simulink model "untitled_2021a"  (R2021a)
settings: Solver=VariableStepAuto  StartTime=0.0  StopTime=inf  RelTol=1e-3
undefined symbols (not defined in the file or in its folder): DiscIntNeverNeededParam
libraries: mobileRoboticsLib x17
settings Model: Creator=its_ghani  LastModifiedBy=nitis

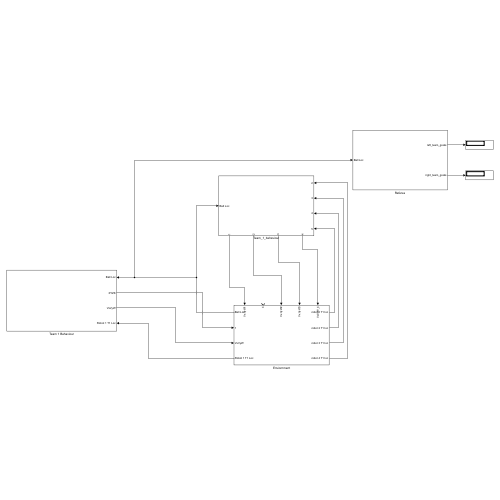
[thumbnail: Simulink's stored preview of the top-level diagram]
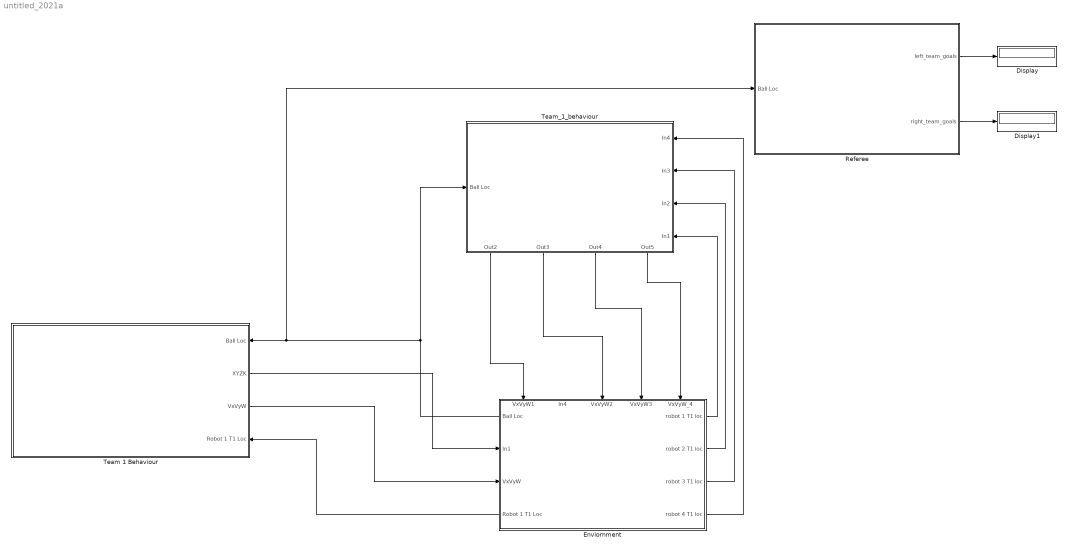
== system untitled_2021a ==
  Display : Display
  Display1 : Display
  Enviornment : Subsystem
      settings: PortSchema="{\"entries\":[{\"content\":{\"sides\":[{\"content\":{\"connectorIds\":[\"Out5\",\"In1\",\"In2\",\"Out6\"]},\"type\":\"ConnectorPlacement.EquallySpacedRectSide\",\"uuid\":\"bfc4f995-18bb-40a5-813e-439d500b4bf9\"},{\"content\":{\"connectorIds\":[\"Out1\",\"Out2\",\"Out3\",\"Out4\"],\"side\":\"RIGHT\"},\"type\":\"ConnectorPlacement.EquallySpacedRectSide\",\"uuid\":\"3fb6b8a6-16df-4a59-8ba5-6321e26d1fdd\"},{\"content\":{\"connectorIds\":[\"In3\",\"In4\",\"In5\",\"In6\",\"In7\"],\"side\":\"TOP\"},\"type\":\"ConnectorPlacement.EquallySpacedRectSide\",\"uuid\":\"a9e4cd1b-3afe-4395-99fa-15aef12a4070\"}]},\"type\":\"ConnectorPlacement.EquallySpacedConnector\",\"uuid\":\"a6ca697e-fe67-43ac-b669-91f3e6c836c9\"}],\"packageUris\":[\"http://schema.mathworks.com/mf0/Connector/R2020b\"],\"version\":\"1.0\"}"
  Referee : Subsystem
  Team 1 Behaviour : Subsystem
      settings: PortSchema="{\"entries\":[{\"content\":{\"sides\":[{\"content\":{\"connectorIds\":[]},\"type\":\"ConnectorPlacement.EquallySpacedRectSide\",\"uuid\":\"be901545-21b9-45e5-bac5-a8cb9027aef5\"},{\"content\":{\"connectorIds\":[\"In1\",\"Out1\",\"Out2\",\"In2\"],\"side\":\"RIGHT\"},\"type\":\"ConnectorPlacement.EquallySpacedRectSide\",\"uuid\":\"b7c1eb84-2f14-4c7f-a74c-d56efbe0743e\"},{\"content\":{\"connectorIds\":[],\"side\":\"TOP\"},\"type\":\"ConnectorPlacement.EquallySpacedRectSide\",\"uuid\":\"aca41723-ed3f-4bd2-8fc1-457d075e3460\"}]},\"type\":\"ConnectorPlacement.EquallySpacedConnector\",\"uuid\":\"e10e22f1-c8f0-4dfc-85d2-4ba01528372d\"}],\"packageUris\":[\"http://schema.mathworks.com/mf0/Connector/R2020b\"],\"version\":\"1.0\"}"
  Team_1_behaviour : Subsystem
      settings: PortSchema="{\"entries\":[{\"content\":{\"sides\":[{\"content\":{\"connectorIds\":[\"In1\"]},\"type\":\"ConnectorPlacement.EquallySpacedRectSide\",\"uuid\":\"3d238569-03e8-47ba-93af-d09e13fdb2d4\"},{\"content\":{\"connectorIds\":[\"In2\",\"In3\",\"In4\",\"In5\"],\"side\":\"RIGHT\"},\"type\":\"ConnectorPlacement.EquallySpacedRectSide\",\"uuid\":\"12d8afb4-4727-4f82-8566-507ab080c6de\"},{\"content\":{\"connectorIds\":[],\"side\":\"TOP\"},\"type\":\"ConnectorPlacement.EquallySpacedRectSide\",\"uuid\":\"c52fa7ec-51b7-43be-84ca-6ce417c012c7\"},{\"content\":{\"connectorIds\":[\"Out1\",\"Out2\",\"Out3\",\"Out4\"],\"side\":\"BOTTOM\"},\"type\":\"ConnectorPlacement.EquallySpacedRectSide\",\"uuid\":\"1ba4ac49-8e90-4b3f-8374-c14756940453\"}]},\"type\":\"ConnectorPlacement.EquallySpacedConnector\",\"uuid\":\"883bb5df-d6b2-498f-94a4-3b94e28c6a8f\"}],\"packageUris\":[\"http://schema.mathworks.com/mf0/Connector/R2020b\"],\"version\":\"1.0\"}"
  wires:
  Enviornment/5(Ball Loc) -> Team_1_behaviour/1(Ball Loc), Referee/1(Ball Loc), Team 1 Behaviour/1(Ball Loc)
  Team 1 Behaviour/1(XYZK) -> Enviornment/1(In1)
  Referee/2(right_team_goals) -> Display1/1
  Referee/1(left_team_goals) -> Display/1
  Team 1 Behaviour/2(VxVyW) -> Enviornment/2(VxVyW)
  Enviornment/6(Robot 1 T1 Loc) -> Team 1 Behaviour/2(Robot 1 T1 Loc)
  Team_1_behaviour/1(Out2) -> Enviornment/3(VxVyW1)
  Team_1_behaviour/2(Out3) -> Enviornment/5(VxVyW2)
  Team_1_behaviour/3(Out4) -> Enviornment/6(VxVyW3)
  Team_1_behaviour/4(Out5) -> Enviornment/7(VxVyW_4)
  Enviornment/1(robot 1 T1 loc) -> Team_1_behaviour/5(In1)
  Enviornment/2(robot 2 T1 loc) -> Team_1_behaviour/4(In2)
  Enviornment/3(robot 3 T1 loc) -> Team_1_behaviour/3(In3)
  Enviornment/4(robot 4 T1 loc) -> Team_1_behaviour/2(In4)

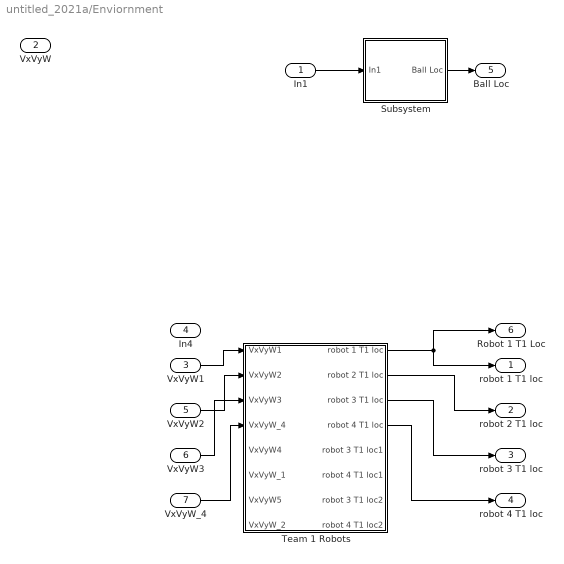
== system untitled_2021a/Enviornment ==
  In1 : Inport
  VxVyW : Inport  Port=2
  VxVyW1 : Inport  Port=3
  In4 : Inport  Port=4
  VxVyW2 : Inport  Port=5
  VxVyW3 : Inport  Port=6
  VxVyW_4 : Inport  Port=7
  "\tTeam 1 Robots" : Subsystem
  Subsystem : Subsystem
  robot 1 T1 loc : Outport
  robot 2 T1 loc : Outport  Port=2
  robot 3 T1 loc : Outport  Port=3
  robot 4 T1 loc : Outport  Port=4
  Ball Loc : Outport  Port=5
  Robot 1 T1 Loc : Outport  Port=6
  wires:
  "\tTeam 1 Robots"/1(robot 1 T1 loc) -> robot 1 T1 loc/1, Robot 1 T1 Loc/1
  "\tTeam 1 Robots"/2(robot 2 T1 loc) -> robot 2 T1 loc/1
  "\tTeam 1 Robots"/3(robot 3 T1 loc) -> robot 3 T1 loc/1
  "\tTeam 1 Robots"/4(robot 4 T1 loc) -> robot 4 T1 loc/1
  VxVyW1/1 -> "\tTeam 1 Robots"/1(VxVyW1)
  VxVyW2/1 -> "\tTeam 1 Robots"/2(VxVyW2)
  VxVyW3/1 -> "\tTeam 1 Robots"/3(VxVyW3)
  VxVyW_4/1 -> "\tTeam 1 Robots"/4(VxVyW_4)
  In1/1 -> Subsystem/1(In1)
  Subsystem/1(Ball Loc) -> Ball Loc/1

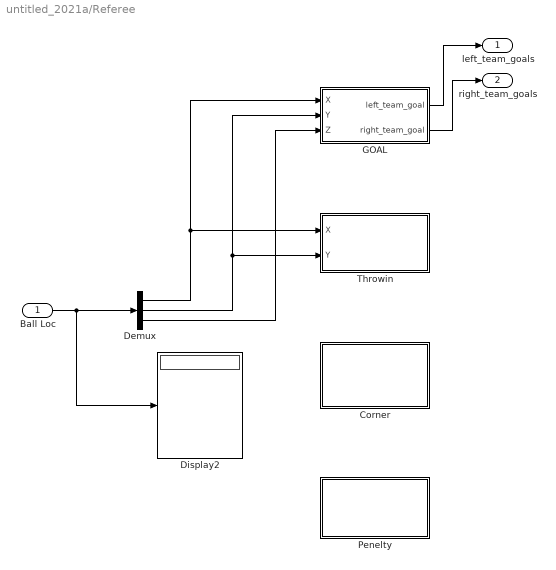
== system untitled_2021a/Referee ==
  Ball Loc : Inport
  Corner : Stateflow chart  TreatAsAtomicUnit=on
  Demux : Demux  Outputs=3
  Display2 : Display
  GOAL : Stateflow chart  TreatAsAtomicUnit=on
  Penelty : Stateflow chart  TreatAsAtomicUnit=on
  Throwin : Stateflow chart  TreatAsAtomicUnit=on
  left_team_goals : Outport
  right_team_goals : Outport  Port=2
  wires:
  Ball Loc/1 -> Display2/1, Demux/1
  Demux/1 -> Throwin/1(X), GOAL/1(X)
  Demux/2 -> Throwin/2(Y), GOAL/2(Y)
  Demux/3 -> GOAL/3(Z)
  GOAL/1(left_team_goal) -> left_team_goals/1
  GOAL/2(right_team_goal) -> right_team_goals/1

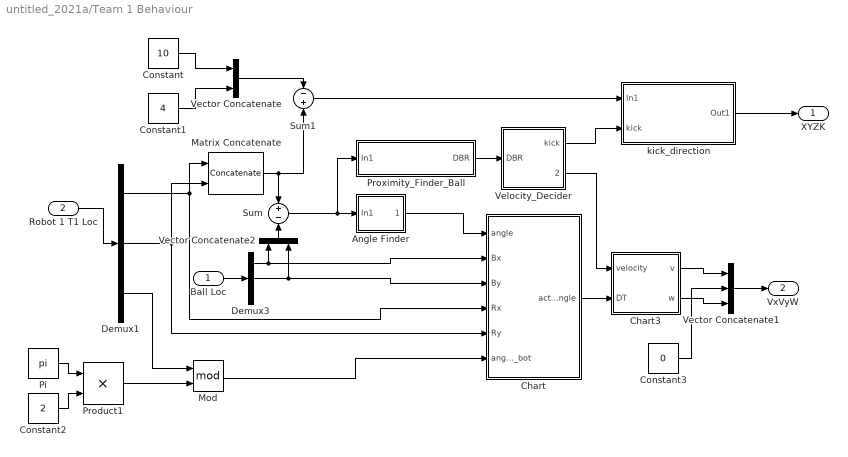
== system untitled_2021a/Team 1 Behaviour ==
  Ball Loc : Inport
  Robot 1 T1 Loc : Inport  Port=2
  Angle Finder : Subsystem
  Chart : Stateflow chart  TreatAsAtomicUnit=on
      settings: PortSchema="{\"entries\":[{\"content\":{\"sides\":[{\"content\":{\"connectorIds\":[\"In5\",\"In1\",\"In2\",\"In3\",\"In4\",\"In6\"]},\"type\":\"ConnectorPlacement.EquallySpacedRectSide\",\"uuid\":\"cd25ea97-6441-4246-83f2-eec847899c89\"},{\"content\":{\"connectorIds\":[\"Out1\"],\"side\":\"RIGHT\"},\"type\":\"ConnectorPlacement.EquallySpacedRectSide\",\"uuid\":\"ef7d77a7-1549-4474-8b84-35bb8af5d0e7\"},{\"content\":{\"connectorIds\":[],\"side\":\"TOP\"},\"type\":\"ConnectorPlacement.EquallySpacedRectSide\",\"uuid\":\"0f0ce596-3061-42ac-890a-62bc4f21ac3e\"},{\"content\":{\"connectorIds\":[],\"side\":\"BOTTOM\"},\"type\":\"ConnectorPlacement.EquallySpacedRectSide\",\"uuid\":\"682b3de5-e999-4954-b7ff-f16ecbf9ea8f\"}]},\"type\":\"ConnectorPlacement.EquallySpacedConnector\",\"uuid\":\"15dca8e2-6a60-4a0d-80a5-3c295a61c828\"}],\"packageUris\":[\"http://schema.mathworks.com/mf0/Connector/R2020b\"],\"version\":\"1.0\"}"
  Chart3 : Stateflow chart  TreatAsAtomicUnit=on
  Constant : Constant  Value=10
  Constant1 : Constant  Value=4
  Constant2 : Constant  Value=2
  Constant3 : Constant  Value=0
  Demux1 : Demux  Outputs=3
  Demux3 : Demux  Outputs=3
  Matrix Concatenate : Concatenate  Mode=Multidimensional array  ConcatenateDimension=2
  Mod : Math  Operator=mod  SaturateOnIntegerOverflow=on
  Pi : Constant  Value=pi  OutDataTypeStr=Inherit: Inherit via back propagation
  Product1 : Product
  Proximity_Finder_Ball : Subsystem
  Sum : Sum  Inputs=+-
  Sum1 : Sum  Inputs=-+
  Vector Concatenate : Concatenate
  Vector Concatenate1 : Concatenate  NumInputs=3
  Vector Concatenate2 : Concatenate
  Velocity_Decider : Stateflow chart  TreatAsAtomicUnit=on
  kick_direction : Subsystem
  XYZK : Outport
  VxVyW : Outport  Port=2
  wires:
  Ball Loc/1 -> Demux3/1
  Sum/1 -> Proximity_Finder_Ball/1(In1), Angle Finder/1(In1)
  Robot 1 T1 Loc/1 -> Demux1/1
  Demux1/1 -> Matrix Concatenate/1, Chart/3(Rx)
  Demux1/2 -> Matrix Concatenate/2, Chart/4(Ry)
  Matrix Concatenate/1 -> Sum1/2, Sum/1
  Demux3/2 -> Vector Concatenate2/2, Chart/2(By)
  Demux3/1 -> Vector Concatenate2/1, Chart/1(Bx)
  Demux1/3 -> Mod/1
  Pi/1 -> Product1/1
  Constant2/1 -> Product1/2
  Product1/1 -> Mod/2
  Chart/1(actual_angle) -> Chart3/2(DT)
  Mod/1 -> Chart/6(angle_bot)
  Angle Finder/1(angle) -> Chart/5(angle)
  Proximity_Finder_Ball/1(DBR) -> Velocity_Decider/1(DBR)
  Velocity_Decider/2(velocity) -> Chart3/1(velocity)
  Constant/1 -> Vector Concatenate/1
  Constant1/1 -> Vector Concatenate/2
  Vector Concatenate/1 -> Sum1/1
  Sum1/1 -> kick_direction/1(In1)
  Velocity_Decider/1(kick) -> kick_direction/2(kick)
  kick_direction/1(Out1) -> XYZK/1
  Chart3/1(v) -> Vector Concatenate1/1
  Chart3/2(w) -> Vector Concatenate1/3
  Constant3/1 -> Vector Concatenate1/2
  Vector Concatenate1/1 -> VxVyW/1
  Vector Concatenate2/1 -> Sum/2

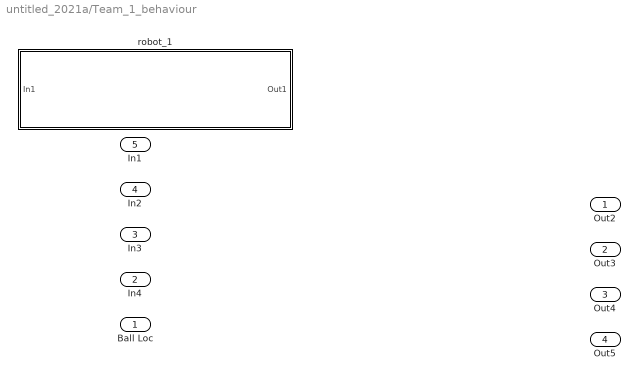
== system untitled_2021a/Team_1_behaviour ==
  Ball Loc : Inport
  In4 : Inport  Port=2
  In3 : Inport  Port=3
  In2 : Inport  Port=4
  In1 : Inport  Port=5
  robot_1 : Subsystem
  Out2 : Outport
  Out3 : Outport  Port=2
  Out4 : Outport  Port=3
  Out5 : Outport  Port=4

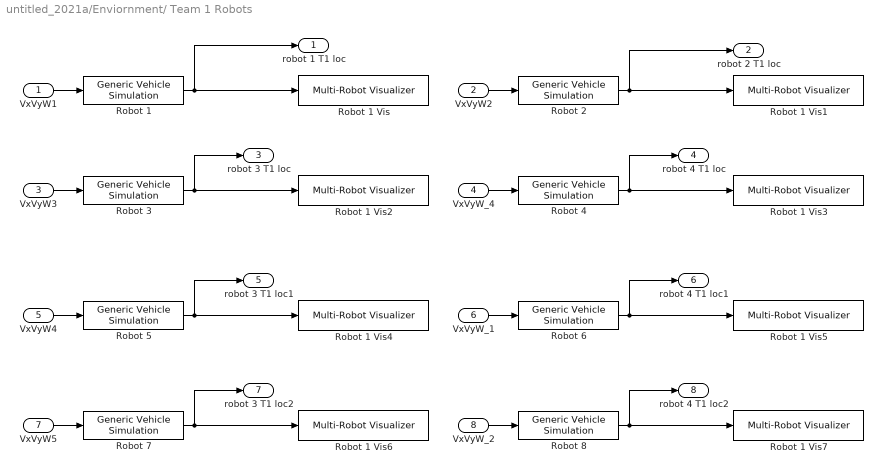
== system untitled_2021a/Enviornment/	Team 1 Robots ==
  VxVyW1 : Inport
  VxVyW2 : Inport  Port=2
  VxVyW3 : Inport  Port=3
  VxVyW_4 : Inport  Port=4
  VxVyW4 : Inport  Port=5
  VxVyW_1 : Inport  Port=6
  VxVyW5 : Inport  Port=7
  VxVyW_2 : Inport  Port=8
  Robot 1 : mobileRoboticsLib/Utilities/Generic Vehicle Simulation  initX=1.5  initY=4  initAngle=0  Ts=0.05
      settings: SourceProductName=Mobile Robotics Simulation Toolbox
  Robot 1 Vis : mobileRoboticsLib/Environments/Multi-Robot Visualizer  idx=1  radius=0.311/2  robotColor=[0 0 1]  showTraj=on  hasLidar=off  sensorOffset=[0,0]  scanAngles=[-pi/4, 0, pi/4]  maxNumScans=0  hasObjDetector=off  objDetectorOffset=[0,0]  objDetectorAngle=0  objDetectorFOV=pi/3  objDetectorMaxRange=5  hasRobotDetector=off  robotDetectorOffset=[0,0]  robotDetectorAngle=0  robotDetectorFOV=pi/3  robotDetectorMaxRange=5  robotDetectorNumDetections=0
      settings: SourceProductName=Mobile Robotics Simulation Toolbox
  Robot 1 Vis1 : mobileRoboticsLib/Environments/Multi-Robot Visualizer  idx=2  radius=0.311/2  robotColor=[0 0 1]  showTraj=on  hasLidar=off  sensorOffset=[0,0]  scanAngles=[-pi/4, 0, pi/4]  maxNumScans=0  hasObjDetector=off  objDetectorOffset=[0,0]  objDetectorAngle=0  objDetectorFOV=pi/3  objDetectorMaxRange=5  hasRobotDetector=off  robotDetectorOffset=[0,0]  robotDetectorAngle=0  robotDetectorFOV=pi/3  robotDetectorMaxRange=5  robotDetectorNumDetections=0
      settings: SourceProductName=Mobile Robotics Simulation Toolbox
  Robot 1 Vis2 : mobileRoboticsLib/Environments/Multi-Robot Visualizer  idx=3  radius=0.311/2  robotColor=[0 0 1]  showTraj=on  hasLidar=off  sensorOffset=[0,0]  scanAngles=[-pi/4, 0, pi/4]  maxNumScans=0  hasObjDetector=off  objDetectorOffset=[0,0]  objDetectorAngle=0  objDetectorFOV=pi/3  objDetectorMaxRange=5  hasRobotDetector=off  robotDetectorOffset=[0,0]  robotDetectorAngle=0  robotDetectorFOV=pi/3  robotDetectorMaxRange=5  robotDetectorNumDetections=0
      settings: SourceProductName=Mobile Robotics Simulation Toolbox
  Robot 1 Vis3 : mobileRoboticsLib/Environments/Multi-Robot Visualizer  idx=4  radius=0.311/2  robotColor=[0 0 1]  showTraj=on  hasLidar=off  sensorOffset=[0,0]  scanAngles=[-pi/4, 0, pi/4]  maxNumScans=0  hasObjDetector=off  objDetectorOffset=[0,0]  objDetectorAngle=0  objDetectorFOV=pi/3  objDetectorMaxRange=5  hasRobotDetector=off  robotDetectorOffset=[0,0]  robotDetectorAngle=0  robotDetectorFOV=pi/3  robotDetectorMaxRange=5  robotDetectorNumDetections=0
      settings: SourceProductName=Mobile Robotics Simulation Toolbox
  Robot 1 Vis4 : mobileRoboticsLib/Environments/Multi-Robot Visualizer  idx=5  radius=0.311/2  robotColor=[1 0 0]  showTraj=on  hasLidar=off  sensorOffset=[0,0]  scanAngles=[-pi/4, 0, pi/4]  maxNumScans=0  hasObjDetector=off  objDetectorOffset=[0,0]  objDetectorAngle=0  objDetectorFOV=pi/3  objDetectorMaxRange=5  hasRobotDetector=off  robotDetectorOffset=[0,0]  robotDetectorAngle=0  robotDetectorFOV=pi/3  robotDetectorMaxRange=5  robotDetectorNumDetections=0
      settings: SourceProductName=Mobile Robotics Simulation Toolbox
  Robot 1 Vis5 : mobileRoboticsLib/Environments/Multi-Robot Visualizer  idx=6  radius=0.311/2  robotColor=[1 0 0]  showTraj=on  hasLidar=off  sensorOffset=[0,0]  scanAngles=[-pi/4, 0, pi/4]  maxNumScans=0  hasObjDetector=off  objDetectorOffset=[0,0]  objDetectorAngle=0  objDetectorFOV=pi/3  objDetectorMaxRange=5  hasRobotDetector=off  robotDetectorOffset=[0,0]  robotDetectorAngle=0  robotDetectorFOV=pi/3  robotDetectorMaxRange=5  robotDetectorNumDetections=0
      settings: SourceProductName=Mobile Robotics Simulation Toolbox
  Robot 1 Vis6 : mobileRoboticsLib/Environments/Multi-Robot Visualizer  idx=7  radius=0.311/2  robotColor=[1 0 0]  showTraj=on  hasLidar=off  sensorOffset=[0,0]  scanAngles=[-pi/4, 0, pi/4]  maxNumScans=0  hasObjDetector=off  objDetectorOffset=[0,0]  objDetectorAngle=0  objDetectorFOV=pi/3  objDetectorMaxRange=5  hasRobotDetector=off  robotDetectorOffset=[0,0]  robotDetectorAngle=0  robotDetectorFOV=pi/3  robotDetectorMaxRange=5  robotDetectorNumDetections=0
      settings: SourceProductName=Mobile Robotics Simulation Toolbox
  Robot 1 Vis7 : mobileRoboticsLib/Environments/Multi-Robot Visualizer  idx=8  radius=0.311/2  robotColor=[1 0 0]  showTraj=on  hasLidar=off  sensorOffset=[0,0]  scanAngles=[-pi/4, 0, pi/4]  maxNumScans=0  hasObjDetector=off  objDetectorOffset=[0,0]  objDetectorAngle=0  objDetectorFOV=pi/3  objDetectorMaxRange=5  hasRobotDetector=off  robotDetectorOffset=[0,0]  robotDetectorAngle=0  robotDetectorFOV=pi/3  robotDetectorMaxRange=5  robotDetectorNumDetections=0
      settings: SourceProductName=Mobile Robotics Simulation Toolbox
  Robot 2 : mobileRoboticsLib/Utilities/Generic Vehicle Simulation  initX=3.25  initY=2.5  initAngle=0  Ts=0.05
      settings: SourceProductName=Mobile Robotics Simulation Toolbox
  Robot 3 : mobileRoboticsLib/Utilities/Generic Vehicle Simulation  initX=3.25  initY=5.5  initAngle=0  Ts=0.05
      settings: SourceProductName=Mobile Robotics Simulation Toolbox
  Robot 4 : mobileRoboticsLib/Utilities/Generic Vehicle Simulation  initX=5.25  initY=4.25  initAngle=0  Ts=0.05
      settings: SourceProductName=Mobile Robotics Simulation Toolbox
  Robot 5 : mobileRoboticsLib/Utilities/Generic Vehicle Simulation  initX=9.5  initY=4  initAngle=pi  Ts=0.05
      settings: SourceProductName=Mobile Robotics Simulation Toolbox
  Robot 6 : mobileRoboticsLib/Utilities/Generic Vehicle Simulation  initX=7.75  initY=4  initAngle=pi  Ts=0.05
      settings: SourceProductName=Mobile Robotics Simulation Toolbox
  Robot 7 : mobileRoboticsLib/Utilities/Generic Vehicle Simulation  initX=7.75  initY=5.5  initAngle=pi  Ts=0.05
      settings: SourceProductName=Mobile Robotics Simulation Toolbox
  Robot 8 : mobileRoboticsLib/Utilities/Generic Vehicle Simulation  initX=7.75  initY=2.5  initAngle=pi  Ts=0.05
      settings: SourceProductName=Mobile Robotics Simulation Toolbox
  robot 1 T1 loc : Outport
  robot 2 T1 loc : Outport  Port=2
  robot 3 T1 loc : Outport  Port=3
  robot 4 T1 loc : Outport  Port=4
  robot 3 T1 loc1 : Outport  Port=5
  robot 4 T1 loc1 : Outport  Port=6
  robot 3 T1 loc2 : Outport  Port=7
  robot 4 T1 loc2 : Outport  Port=8
  wires:
  Robot 1/1 -> robot 1 T1 loc/1, Robot 1 Vis/1
  VxVyW1/1 -> Robot 1/1
  VxVyW2/1 -> Robot 2/1
  Robot 2/1 -> robot 2 T1 loc/1, Robot 1 Vis1/1
  Robot 3/1 -> Robot 1 Vis2/1, robot 3 T1 loc/1
  VxVyW3/1 -> Robot 3/1
  VxVyW_4/1 -> Robot 4/1
  Robot 4/1 -> robot 4 T1 loc/1, Robot 1 Vis3/1
  VxVyW4/1 -> Robot 5/1
  Robot 5/1 -> robot 3 T1 loc1/1, Robot 1 Vis4/1
  Robot 6/1 -> Robot 1 Vis5/1, robot 4 T1 loc1/1
  VxVyW_1/1 -> Robot 6/1
  Robot 7/1 -> Robot 1 Vis6/1, robot 3 T1 loc2/1
  VxVyW5/1 -> Robot 7/1
  VxVyW_2/1 -> Robot 8/1
  Robot 8/1 -> robot 4 T1 loc2/1, Robot 1 Vis7/1

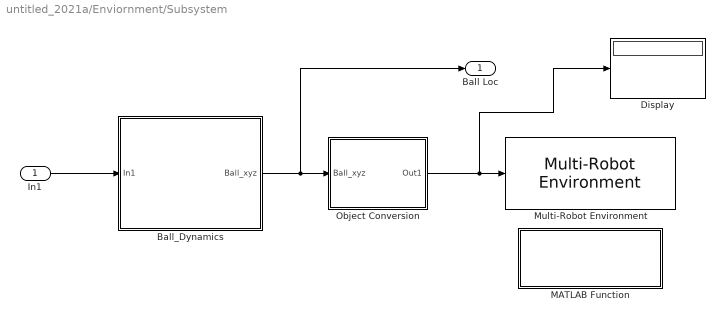
== system untitled_2021a/Enviornment/Subsystem ==
  In1 : Inport
  Ball_Dynamics : Subsystem
  Display : Display
  MATLAB Function : MATLAB Function  TreatAsAtomicUnit=on
  Multi-Robot Environment : mobileRoboticsLib/Environments/Multi-Robot Environment  numRobots=8  showWaypoints=off  showObjects=on  objectColors=[1 0 0]  objectMarkers='C'  showRobotIds=on  plotSensorLines=on
      settings: SourceProductName=Mobile Robotics Simulation Toolbox
  Object Conversion : Subsystem
  Ball Loc : Outport
  wires:
  Object Conversion/1(Out1) -> Multi-Robot Environment/1, Display/1
  Ball_Dynamics/1(Ball_xyz) -> Ball Loc/1, Object Conversion/1(Ball_xyz)
  In1/1 -> Ball_Dynamics/1(In1)

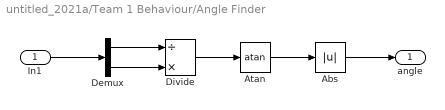
== system untitled_2021a/Team 1 Behaviour/Angle Finder ==
  In1 : Inport
  Abs : Abs
  Atan : Trigonometry  Operator=atan
  Demux : Demux  Outputs=2
  Divide : Product  Inputs=/*
  angle : Outport
  wires:
  Divide/1 -> Atan/1
  Demux/2 -> Divide/2
  Demux/1 -> Divide/1
  Atan/1 -> Abs/1
  Abs/1 -> angle/1
  In1/1 -> Demux/1

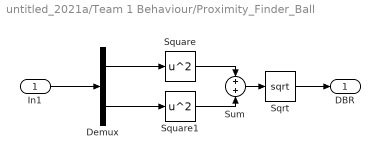
== system untitled_2021a/Team 1 Behaviour/Proximity_Finder_Ball ==
  In1 : Inport
  Demux : Demux  Outputs=2
  Sqrt : Sqrt  SaturateOnIntegerOverflow=on
  Square : Math  Operator=square  SaturateOnIntegerOverflow=on
  Square1 : Math  Operator=square  SaturateOnIntegerOverflow=on
  Sum : Sum
  DBR : Outport
  wires:
  In1/1 -> Demux/1
  Demux/1 -> Square/1
  Demux/2 -> Square1/1
  Square1/1 -> Sum/2
  Square/1 -> Sum/1
  Sum/1 -> Sqrt/1
  Sqrt/1 -> DBR/1

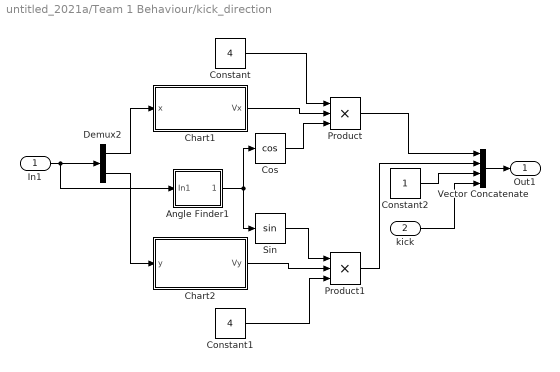
== system untitled_2021a/Team 1 Behaviour/kick_direction ==
  In1 : Inport
  kick : Inport  Port=2
  Angle Finder1 : Subsystem
  Chart1 : Stateflow chart  TreatAsAtomicUnit=on
  Chart2 : Stateflow chart  TreatAsAtomicUnit=on
  Constant : Constant  Value=4
  Constant1 : Constant  Value=4
  Constant2 : Constant
  Cos : Trigonometry  Operator=cos
  Demux2 : Demux  Outputs=2
  Product : Product  Inputs=3
  Product1 : Product  Inputs=3
  Sin : Trigonometry
  Vector Concatenate : Concatenate  NumInputs=4
  Out1 : Outport
  wires:
  Demux2/2 -> Chart2/1(y)
  Demux2/1 -> Chart1/1(x)
  In1/1 -> Angle Finder1/1(In1), Demux2/1
  Chart1/1(Vx) -> Product/2
  Cos/1 -> Product/3
  Angle Finder1/1(angle) -> Cos/1, Sin/1
  Constant/1 -> Product/1
  Constant1/1 -> Product1/3
  Chart2/1(Vy) -> Product1/2
  Sin/1 -> Product1/1
  Product/1 -> Vector Concatenate/1
  Product1/1 -> Vector Concatenate/2
  Constant2/1 -> Vector Concatenate/3
  kick/1 -> Vector Concatenate/4
  Vector Concatenate/1 -> Out1/1

== system untitled_2021a/Team_1_behaviour/robot_1 ==
  In1 : Inport
  Out1 : Outport
  wires:
  In1/1 -> Out1/1

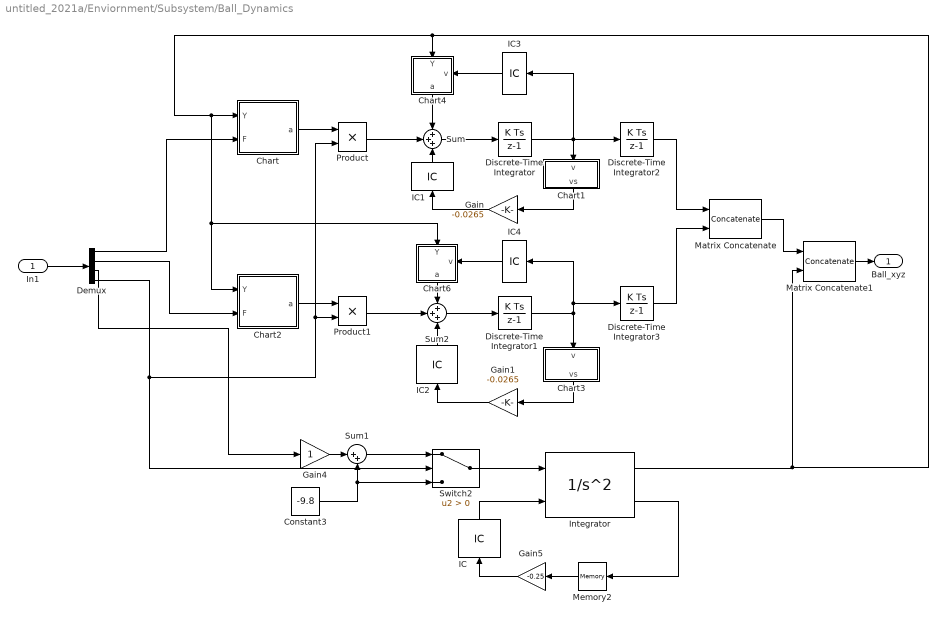
== system untitled_2021a/Enviornment/Subsystem/Ball_Dynamics ==
  In1 : Inport
  Chart : Stateflow chart  TreatAsAtomicUnit=on
  Chart1 : Stateflow chart  TreatAsAtomicUnit=on
      settings: PortSchema="{\"entries\":[{\"content\":{\"sides\":[{\"content\":{\"connectorIds\":[]},\"type\":\"ConnectorPlacement.EquallySpacedRectSide\",\"uuid\":\"edcb69b6-c92b-474e-86d7-1e52c2e82b28\"},{\"content\":{\"connectorIds\":[],\"side\":\"RIGHT\"},\"type\":\"ConnectorPlacement.EquallySpacedRectSide\",\"uuid\":\"df9771e4-6870-4305-9c84-3f71fcb76e6b\"},{\"content\":{\"connectorIds\":[\"In1\"],\"side\":\"TOP\"},\"type\":\"ConnectorPlacement.EquallySpacedRectSide\",\"uuid\":\"56b80241-156d-4669-9174-884a577f2013\"},{\"content\":{\"connectorIds\":[\"Out1\"],\"side\":\"BOTTOM\"},\"type\":\"ConnectorPlacement.EquallySpacedRectSide\",\"uuid\":\"179af6a7-cab5-4faa-a562-268e2d2e4d3e\"}]},\"type\":\"ConnectorPlacement.EquallySpacedConnector\",\"uuid\":\"707001f1-02b8-4f5e-ba3f-f155c99072e5\"}],\"packageUris\":[\"http://schema.mathworks.com/mf0/Connector/R2020b\"],\"version\":\"1.0\"}"
  Chart2 : Stateflow chart  TreatAsAtomicUnit=on
  Chart3 : Stateflow chart  TreatAsAtomicUnit=on
      settings: PortSchema="{\"entries\":[{\"content\":{\"sides\":[{\"content\":{\"connectorIds\":[]},\"type\":\"ConnectorPlacement.EquallySpacedRectSide\",\"uuid\":\"edcb69b6-c92b-474e-86d7-1e52c2e82b28\"},{\"content\":{\"connectorIds\":[],\"side\":\"RIGHT\"},\"type\":\"ConnectorPlacement.EquallySpacedRectSide\",\"uuid\":\"df9771e4-6870-4305-9c84-3f71fcb76e6b\"},{\"content\":{\"connectorIds\":[\"In1\"],\"side\":\"TOP\"},\"type\":\"ConnectorPlacement.EquallySpacedRectSide\",\"uuid\":\"56b80241-156d-4669-9174-884a577f2013\"},{\"content\":{\"connectorIds\":[\"Out1\"],\"side\":\"BOTTOM\"},\"type\":\"ConnectorPlacement.EquallySpacedRectSide\",\"uuid\":\"179af6a7-cab5-4faa-a562-268e2d2e4d3e\"}]},\"type\":\"ConnectorPlacement.EquallySpacedConnector\",\"uuid\":\"707001f1-02b8-4f5e-ba3f-f155c99072e5\"}],\"packageUris\":[\"http://schema.mathworks.com/mf0/Connector/R2020b\"],\"version\":\"1.0\"}"
  Chart4 : Stateflow chart  TreatAsAtomicUnit=on
      settings: PortSchema="{\"entries\":[{\"content\":{\"sides\":[{\"content\":{\"connectorIds\":[]},\"type\":\"ConnectorPlacement.EquallySpacedRectSide\",\"uuid\":\"edcb69b6-c92b-474e-86d7-1e52c2e82b28\"},{\"content\":{\"connectorIds\":[\"In2\"],\"side\":\"RIGHT\"},\"type\":\"ConnectorPlacement.EquallySpacedRectSide\",\"uuid\":\"df9771e4-6870-4305-9c84-3f71fcb76e6b\"},{\"content\":{\"connectorIds\":[\"In1\"],\"side\":\"TOP\"},\"type\":\"ConnectorPlacement.EquallySpacedRectSide\",\"uuid\":\"56b80241-156d-4669-9174-884a577f2013\"},{\"content\":{\"connectorIds\":[\"Out1\"],\"side\":\"BOTTOM\"},\"type\":\"ConnectorPlacement.EquallySpacedRectSide\",\"uuid\":\"6d9abc99-74e1-40c2-a49f-e0d9410a29cc\"}]},\"type\":\"ConnectorPlacement.EquallySpacedConnector\",\"uuid\":\"707001f1-02b8-4f5e-ba3f-f155c99072e5\"}],\"packageUris\":[\"http://schema.mathworks.com/mf0/Connector/R2020b\"],\"version\":\"1.0\"}"
  Chart6 : Stateflow chart  TreatAsAtomicUnit=on
      settings: PortSchema="{\"entries\":[{\"content\":{\"sides\":[{\"content\":{\"connectorIds\":[]},\"type\":\"ConnectorPlacement.EquallySpacedRectSide\",\"uuid\":\"edcb69b6-c92b-474e-86d7-1e52c2e82b28\"},{\"content\":{\"connectorIds\":[\"In2\"],\"side\":\"RIGHT\"},\"type\":\"ConnectorPlacement.EquallySpacedRectSide\",\"uuid\":\"df9771e4-6870-4305-9c84-3f71fcb76e6b\"},{\"content\":{\"connectorIds\":[\"In1\"],\"side\":\"TOP\"},\"type\":\"ConnectorPlacement.EquallySpacedRectSide\",\"uuid\":\"56b80241-156d-4669-9174-884a577f2013\"},{\"content\":{\"connectorIds\":[\"Out1\"],\"side\":\"BOTTOM\"},\"type\":\"ConnectorPlacement.EquallySpacedRectSide\",\"uuid\":\"6d9abc99-74e1-40c2-a49f-e0d9410a29cc\"}]},\"type\":\"ConnectorPlacement.EquallySpacedConnector\",\"uuid\":\"707001f1-02b8-4f5e-ba3f-f155c99072e5\"}],\"packageUris\":[\"http://schema.mathworks.com/mf0/Connector/R2020b\"],\"version\":\"1.0\"}"
  Constant3 : Constant  Value=-9.8
  Demux : Demux
  Discrete-Time Integrator : DiscreteIntegrator  SampleTime=-1  ICPrevOutput=DiscIntNeverNeededParam  ICPrevScaledInput=DiscIntNeverNeededParam
  Discrete-Time Integrator1 : DiscreteIntegrator  SampleTime=-1  ICPrevOutput=DiscIntNeverNeededParam  ICPrevScaledInput=DiscIntNeverNeededParam
  Discrete-Time Integrator2 : DiscreteIntegrator  InitialCondition=5.5  SampleTime=-1  ICPrevOutput=DiscIntNeverNeededParam  ICPrevScaledInput=DiscIntNeverNeededParam
  Discrete-Time Integrator3 : DiscreteIntegrator  InitialCondition=4  SampleTime=-1  ICPrevOutput=DiscIntNeverNeededParam  ICPrevScaledInput=DiscIntNeverNeededParam
  Gain : Gain  Gain=-0.0265
  Gain1 : Gain  Gain=-0.0265
  Gain4 : Gain
  Gain5 : Gain  Gain=-0.25
  IC : InitialCondition
  IC{1..4} (4 alike) : InitialCondition  Value=0
  Integrator : SecondOrderIntegrator  ICX=0  LimitX=on  LowerLimitX=0.0  StateNameX='Position'  ICSourceDXDT=external  StateNameDXDT='Velocity'  ReinitDXDTwhenXreachesSaturation=on
  Matrix Concatenate : Concatenate  Mode=Multidimensional array  ConcatenateDimension=2
  Matrix Concatenate1 : Concatenate  Mode=Multidimensional array  ConcatenateDimension=2
  Memory2 : Memory
  Product : Product
  Product1 : Product
  Sum : Sum  Inputs=+++
  Sum1 : Sum  Inputs=|++
  Sum2 : Sum  Inputs=+++
  Switch2 : Switch  Criteria=u2 > Threshold
  Ball_xyz : Outport
  wires:
  Constant3/1 -> Sum1/2, Switch2/3
  Integrator/2 -> Memory2/1
  Memory2/1 -> Gain5/1
  IC/1 -> Integrator/2
  Switch2/1 -> Integrator/1
  Sum1/1 -> Switch2/1
  Gain4/1 -> Sum1/1
  Matrix Concatenate/1 -> Matrix Concatenate1/1
  Matrix Concatenate1/1 -> Ball_xyz/1
  Demux/3 -> Gain4/1
  Demux/4 -> Switch2/2, Product/2, Product1/2
  Gain5/1 -> IC/1
  In1/1 -> Demux/1
  Gain/1 -> IC1/1
  Chart/1(a) -> Product/1
  Sum/1 -> Discrete-Time Integrator/1
  Discrete-Time Integrator1/1 -> IC4/1, Discrete-Time Integrator3/1, Chart3/1(v)
  Chart2/1(a) -> Product1/1
  Gain1/1 -> IC2/1
  Product1/1 -> Sum2/2
  Sum2/1 -> Discrete-Time Integrator1/1
  Demux/1 -> Chart/2(F)
  Demux/2 -> Chart2/2(F)
  Discrete-Time Integrator2/1 -> Matrix Concatenate/1
  Discrete-Time Integrator3/1 -> Matrix Concatenate/2
  Integrator/1 -> Chart6/1(Y), Chart2/1(Y), Chart/1(Y), Chart4/1(Y), Matrix Concatenate1/2
  Chart1/1(vs) -> Gain/1
  Chart3/1(vs) -> Gain1/1
  IC3/1 -> Chart4/2(v)
  Discrete-Time Integrator/1 -> IC3/1, Discrete-Time Integrator2/1, Chart1/1(v)
  Product/1 -> Sum/2
  IC2/1 -> Sum2/3
  IC1/1 -> Sum/3
  IC4/1 -> Chart6/2(v)
  Chart4/1(a) -> Sum/1
  Chart6/1(a) -> Sum2/1

== system untitled_2021a/Enviornment/Subsystem/Object Conversion ==
  Ball_xyz : Inport
  Constant : Constant
  Demux : Demux  Outputs=3
  Matrix Concatenate : Concatenate  NumInputs=3  Mode=Multidimensional array
  Out1 : Outport
  wires:
  Ball_xyz/1 -> Demux/1
  Matrix Concatenate/1 -> Out1/1
  Demux/1 -> Matrix Concatenate/1
  Demux/2 -> Matrix Concatenate/2
  Constant/1 -> Matrix Concatenate/3

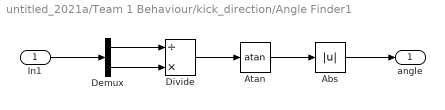
== system untitled_2021a/Team 1 Behaviour/kick_direction/Angle Finder1 ==
  In1 : Inport
  Abs : Abs
  Atan : Trigonometry  Operator=atan
  Demux : Demux  Outputs=2
  Divide : Product  Inputs=/*
  angle : Outport
  wires:
  Divide/1 -> Atan/1
  Demux/2 -> Divide/2
  Demux/1 -> Divide/1
  Atan/1 -> Abs/1
  Abs/1 -> angle/1
  In1/1 -> Demux/1

== stateflow chart untitled_2021a/Referee/Throwin ==
  data: X input; Y input

== stateflow chart untitled_2021a/Referee/Corner ==

== stateflow chart untitled_2021a/Referee/Penelty ==

== matlab function untitled_2021a/Enviornment/Subsystem/MATLAB Function ==

function plotEnvironment

coder.extrinsic('evalin');
persistent hasPlotted
if isempty(hasPlotted)
    evalin('base','environment_Plot');
    hasPlotted = true;
end

== stateflow chart untitled_2021a/Enviornment/Subsystem/Ball_Dynamics/Chart ==
  state on_ground
    du:
    if(abs(F)>2.6)
    a = (abs(F)-2.6) * (F/abs(F)) / 0.43
    else
    a = 0
    end
  state off_ground
    du:
    a = F/0.43
  (default) -> on_ground
  off_ground -> on_ground : [Y ==0]
  on_ground -> off_ground : [Y > 0]
  data: Y input; F input; a output

== stateflow chart untitled_2021a/Enviornment/Subsystem/Ball_Dynamics/Chart1 ==
  state calculations_neg
    du:
    vs = (abs(v))*(abs(v))*(-1)
  state calculations_pos
    du:
    vs = v*v
  (default) -> calculations_neg
  calculations_pos -> calculations_neg : [v<0]
  calculations_neg -> calculations_pos : [v>0]
  data: vs output; v input

== stateflow chart untitled_2021a/Enviornment/Subsystem/Ball_Dynamics/Chart2 ==
  state on_ground
    du:
    if(abs(F)>2.6)
    a = (abs(F) - 2.6) * (F/abs(F)) / 0.43
    else
    a = 0
    end
  state off_ground
    du:
    a = F/0.43
  (default) -> on_ground
  off_ground -> on_ground : [Y ==0]
  on_ground -> off_ground : [Y > 0]
  data: Y input; F input; a output

== stateflow chart untitled_2021a/Enviornment/Subsystem/Ball_Dynamics/Chart3 ==
  state calculations_neg
    du:
    vs = (abs(v))*(abs(v))*(-1)
  state calculations_pos
    du:
    vs = v*v
  (default) -> calculations_neg
  calculations_pos -> calculations_neg : [v<0]
  calculations_neg -> calculations_pos : [v>=0]
  data: vs output; v input

== stateflow chart untitled_2021a/Enviornment/Subsystem/Ball_Dynamics/Chart4 ==
  state in_motion
    du:
    if (v > 0)
    a = -(0.32*0.98)
    else if(v<0)
    a = (0.32*0.98)
    end
    end
  state stationary
    du:
    a = 0;
  (default) -> in_motion
  in_motion -> stationary : [abs(v) < 0.03 | Y>0]
  stationary -> in_motion : [abs(v)>0.03]
  data: Y input; a output; v input

== stateflow chart untitled_2021a/Enviornment/Subsystem/Ball_Dynamics/Chart6 ==
  state in_motion
    du:
    if (v > 0)
    a = -(0.32*0.98)
    else if(v<0)
    a = (0.32*0.98)
    end
    end
  state stationary
    du:
    a = 0;
  (default) -> in_motion
  in_motion -> stationary : [abs(v) < 0.01 | Y>0]
  stationary -> in_motion : [abs(v)>0.02]
  data: Y input; a output; v input

== stateflow chart untitled_2021a/Team 1 Behaviour/kick_direction/Chart1 ==
  state x_pos
    du:
    Vx = 1
  state x_neg
    du:
    Vx = -1
  (default) -> x_pos
  x_pos -> x_neg : [x > 0]
  x_neg -> x_pos : [x<1]
  data: Vx output; x input

== stateflow chart untitled_2021a/Team 1 Behaviour/kick_direction/Chart2 ==
  state y_pos
    du:
    Vy = 1
  state y_neg
    du:
    Vy = -1
  (default) -> y_pos
  y_pos -> y_neg : [y > 0]
  y_neg -> y_pos : [y<1]
  data: y input; Vy output

== stateflow chart untitled_2021a/Team 1 Behaviour/Velocity_Decider ==
  state Robot_Far
    du:
    velocity = 1;
    kick = 0;
  state Robot_Close
    du:
    velocity = 0;
    kick = 1;
  (default) -> Robot_Far
  Robot_Far -> Robot_Close : [DBR <= 0.25]
  Robot_Close -> Robot_Far : [DBR > 0.25]
  data: kick output; DBR input; velocity output

== stateflow chart untitled_2021a/Team 1 Behaviour/Chart ==
  state second_coordinate
    du:
    actual_angle = -pi +angle + angle_bot;
  state first_coordinate
    du:
    actual_angle = angle_bot - angle;
  state ffourth_coordinate
    du:
    actual_angle = -(2*pi) + angle + angle_bot
  state Third_coordinate
    du:
    actual_angle =-(pi) - angle + angle_bot;
  (default) -> first_coordinate
  first_coordinate -> second_coordinate [order 1] : [ Rx>Bx && Ry<By ]
  second_coordinate -> first_coordinate [order 1] : [ Rx<Bx && Ry<By]
  ffourth_coordinate -> second_coordinate [order 1] : [ Rx>Bx && Ry<By ]
  first_coordinate -> Third_coordinate [order 3] : [ Rx>Bx && Ry>By]
  second_coordinate -> Third_coordinate [order 3] : [ Rx>Bx && Ry>By ]
  Third_coordinate -> second_coordinate [order 1] : [ Rx>Bx && Ry<By ]
  second_coordinate -> ffourth_coordinate [order 2] : [ Rx<Bx && Ry>By ]
  Third_coordinate -> first_coordinate [order 2] : [ Rx<Bx && Ry<By ]
  ffourth_coordinate -> first_coordinate [order 2] : [ Rx<Bx && Ry<By ]
  first_coordinate -> ffourth_coordinate [order 2] : [ Rx<Bx && Ry>By ]
  Third_coordinate -> ffourth_coordinate [order 3] : [ Rx<Bx && Ry>By ]
  ffourth_coordinate -> Third_coordinate [order 3] : [ Rx>Bx && Ry>By]
  data: Bx input; By input; Rx input; Ry input; angle input; actual_angle output; angle_bot input

== stateflow chart untitled_2021a/Team 1 Behaviour/Chart3 ==
  state stop
    du:
    w = 0;
    v=0.25 * velocity;
  state RCW
    du:
    w = -1*1;
    v=0;
  state RCCW
    du:
    w =1*1;
    v=0;
  (default) -> stop
  stop -> RCCW [order 2] : [after(1,sec) && DT > 0]
  stop -> RCW [order 1] : [after(1,sec) && DT < 0]
  RCW -> stop [order 1] : [DT<= 0.1 && DT>= -0.1]
  RCCW -> stop [order 1] : [DT<= 0.1 && DT>= -0.1]
  RCCW -> RCW [order 2] : [DT>0]
  RCW -> RCCW [order 2] : [DT<0]
  data: velocity input; v output; DT input; w output

== stateflow chart untitled_2021a/Referee/GOAL ==
  state Start
    en:
    right_team_goal = 0;
    left_team_goal = 0;
  state Goal_left
    en:
    right_team_goal = right_team_goal +1 ;
  state in_field
    en:
  state Goal_right
    en:
    left_team_goal = left_team_goal + 1;
  (default) -> Start
  Start -> in_field : [X > 1 && X<10 && Y > 1  && Y < 7]
  in_field -> Goal_left [order 2] : [fix(X) == 1 && Y > 2.7  && Y < 5.3 && Z < 1.2]
  Goal_right -> in_field : [X > 1 && X<10 && Y > 1  && Y < 7]
  in_field -> Goal_right [order 1] : [fix(X) == 10 && Y > 2.7  && Y < 5.3 && Z <1.2]
  Goal_left -> in_field : [X > 1 && X<10 && Y > 1  && Y < 7]
  data: X input; Y input; Z input; left_team_goal output; right_team_goal output
